simulink model "exampleKinematicViscosity2"  (R2018b)
settings: Solver=FixedStepDiscrete  StartTime=0.0  StopTime=10  FixedStep=1  RelTol=1e-3  EnableMultiTasking=on
libraries: carnot x3
settings Model: Creator=awohlfei  LastModifiedBy=drhf
settings DataIOCC: LimitDataPoints=on  SaveFormat=Array  SignalLoggingSaveFormat=ModelDataLogs
settings OptimizationCC: ExpressionDepthLimit=2147483647  LifeSpan=inf
settings DebuggingCC: UnderspecifiedInitializationDetection=Classic  MergeDetectMultiDrivingBlocksExec=none  SolverPrmCheckMsg=warning  StateNameClashWarn=warning  SFUnexpectedBacktrackingDiag=warning  SFNoUnconditionalDefaultTransitionDiag=warning  SFExecutionAtInitializationDiag=none
settings HardwareCC: ProdBitPerPointer=32  ProdBitPerSizeT=32  ProdBitPerPtrDiffT=32  ProdLargestAtomicFloat=None  ProdIntDivRoundTo=Undefined  ProdEndianess=Unspecified  ProdWordSize=32  ProdHWDeviceType=32-bit Generic
settings ModelReferenceCC: PropagateSignalLabelsOutOfModel=off
settings SFSimCC: SimUseLocalCustomCode=off
settings RTWCC: RTWUseLocalCustomCode=off
settings CodeAppCC: StateflowObjectComments=on
settings GRTTargetCC: TargetLangStandard=C89/C90 (ANSI)  GeneratePreprocessorConditionals=Disable all
settings ConfigComp: CovMetricSettings=dw  CovHtmlReporting=on  CovSaveCumulativeToWorkspaceVar=on  CovSaveSingleToWorkspaceVar=on  CovExternalEMLEnable=off

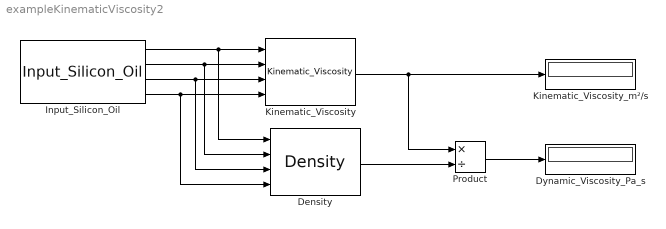
== system exampleKinematicViscosity2 ==
  Density : carnot/Basic/Material_Properties/Density  VariantControl=CarlibClassic  INPUTARGUMENTS=state variables (classic)  DEBUGLEVEL=DEBUGLEVEL  MAXTOTALWARNINGS=inf  MAXCONSECUTIVEWARNINGS=inf  WRITETOFILE=0  FILENAME='errors.txt'
  Dynamic_Viscosity_Pa_s : Display
  Input_Silicon_Oil : carnot/Basic/Material_Properties/Input_Silicon_Oil  T=50  p=1e5
  Kinematic_Viscosity : carnot/Basic/Material_Properties/Kinematic_Viscosity  VariantControl=CarlibClassic  INPUTARGUMENTS=state variables (classic)  DEBUGLEVEL=WARNINGLEVEL  MAXTOTALMESSAGES=inf  MAXCONSECUTIVEMESSAGES=inf  WRITETOFILE=0  FILENAME='errors.txt'
  Kinematic_Viscosity_m²/s : Display
  Product : Product  Inputs=*/
  wires:
  Kinematic_Viscosity/1 -> Product/1, Kinematic_Viscosity_m²/s/1
  Input_Silicon_Oil/1 -> Kinematic_Viscosity/1, Density/1
  Input_Silicon_Oil/2 -> Kinematic_Viscosity/2, Density/2
  Input_Silicon_Oil/4 -> Kinematic_Viscosity/4, Density/4
  Input_Silicon_Oil/3 -> Kinematic_Viscosity/3, Density/3
  Density/1 -> Product/2
  Product/1 -> Dynamic_Viscosity_Pa_s/1
